simulink model "shortcircuit"  (Simulink 7.6)
settings: Solver=ode45  StartTime=0.0  StopTime=0.2  RelTol=1e-3
libraries: powerlib x10
settings Model: Creator=Martine  LastModifiedBy=ROOTS

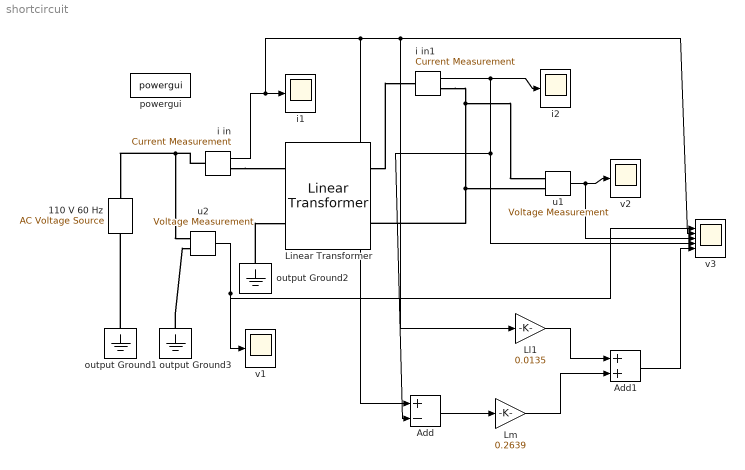
== system shortcircuit ==
  110 V 60 Hz : powerlib/Electrical Sources/AC Voltage Source  Description=source block  DialogController=POWERSYS.PowerSysDialog  SystemSampleTime=-1  Amplitude=155.563  Phase=0  Frequency=60  SampleTime=0  Measurements=None
      settings: AttributesFormatString=\n
  Add : Sum  Inputs=+-
  Add1 : Sum
  Linear Transformer : powerlib/Elements/Linear Transformer  DialogController=POWERSYS.PowerSysDialog  PhysicalDomain=powersysdomain  SubClassName=unknown  LeftPortType=p1  RightPortType=p1  LConnTagsString=a|b  RConnTagsString=A|B  UNITS=SI  NominalPower=[75e3,60]  winding1=[110 6 0.0135]  winding2=[110 5 0.0135]  ThreeWindings=off  winding3=[120 0.00384 0]  RmLm=[99.5 0.2639]  Measurements=None  DataType=on
  Ll1 : Gain  Gain=0.0135
  Lm : Gain  Gain=0.2639
  i in : powerlib/Measurements/Current Measurement  Tag=PoWeRsYsTeMmEaSuReMeNt  DialogController=POWERSYS.PowerSysDialog  SystemSampleTime=-1  PhasorSimulation=off  OutputType=Magnitude  PSBequivalent=0
  i in1 : powerlib/Measurements/Current Measurement  Tag=PoWeRsYsTeMmEaSuReMeNt  DialogController=POWERSYS.PowerSysDialog  SystemSampleTime=-1  PhasorSimulation=off  OutputType=Magnitude  PSBequivalent=0
  i1 : Scope
      settings: DeleteFcn=simscope BlockIsBeingDestroyed  PostSaveFcn=simscope Save  TickLabels=on  TimeRange=0.1  YMin=-10  YMax=10  SaveName=ScopeData3  DataFormat=Array
  i2 : Scope
      settings: DeleteFcn=simscope BlockIsBeingDestroyed  PostSaveFcn=simscope Save  TickLabels=on  TimeRange=0.1  YMin=-12.5  YMax=12.5  SaveName=ScopeData2  DataFormat=Array
  output Ground1 : powerlib/Elements/Ground  DialogController=POWERSYS.PowerSysDialog  PhysicalDomain=powersysdomain  SubClassName=unknown  LeftPortType=p1  RightPortType=p1  LConnTagsString=a
  output Ground2 : powerlib/Elements/Ground  DialogController=POWERSYS.PowerSysDialog  PhysicalDomain=powersysdomain  SubClassName=unknown  LeftPortType=p1  RightPortType=p1  LConnTagsString=a
  output Ground3 : powerlib/Elements/Ground  DialogController=POWERSYS.PowerSysDialog  PhysicalDomain=powersysdomain  SubClassName=unknown  LeftPortType=p1  RightPortType=p1  LConnTagsString=a
  powergui : powerlib/powergui  SystemSampleTime=-1  SimulationMode=Continuous  SampleTime=0  frequency=60  SPID=off  DisableSnubberDevices=off  DisableRonSwitches=off  DisableVfSwitches=off  SwTol=0  Interpol=off  frequencyindice=60  echomessages=off  HookPort=off  DisplayEquations=off  FunctionMessages=off  EnableUseOfTLC=off  x0status=blocks  RestoreLinks=warning  ResistiveCurrentMeasurement=off  Frange=[0:2:500]  Ylog=off  Xlog=on  ShowGrid=off  save=off  variable=ZData  ZoomFFT=on  StartTime=0.0  cycles=1  DisplayStyle=1  fundamental=60  FreqAxis=off  MaxFrequency=1000  frequencyindicesteady=1  RmsSteady=1  display=off  Ts=0  methode=off
  u1 : powerlib/Measurements/Voltage Measurement  Tag=PoWeRsYsTeMmEaSuReMeNt  DialogController=POWERSYS.PowerSysDialog  SystemSampleTime=-1  PhasorSimulation=off  OutputType=Magnitude  PSBequivalent=0
  u2 : powerlib/Measurements/Voltage Measurement  Tag=PoWeRsYsTeMmEaSuReMeNt  DialogController=POWERSYS.PowerSysDialog  SystemSampleTime=-1  PhasorSimulation=off  OutputType=Magnitude  PSBequivalent=0
  v1 : Scope
      settings: DeleteFcn=simscope BlockIsBeingDestroyed  PostSaveFcn=simscope Save  TickLabels=on  TimeRange=0.1  YMin=-200  YMax=200  DataFormat=Array
  v2 : Scope
      settings: DeleteFcn=simscope BlockIsBeingDestroyed  PostSaveFcn=simscope Save  TickLabels=on  TimeRange=0.1  YMin=-200  YMax=200  DataFormat=Array
  v3 : Scope  NumInputPorts=5
      settings: DeleteFcn=simscope BlockIsBeingDestroyed  PostSaveFcn=simscope Save  TickLabels=on  TimeRange=0.2  YMin=-200~-5~-5~-20~-5  YMax=200~5~5~20~5  SaveName=ScopeData4  DataFormat=Array
  wires:
  i in/1 -> i1/1, Add/1, v3/2, Ll1/1
  u1/1 -> v2/1, v3/3
  u2/1 -> v1/1, v3/1
  i in1/1 -> i2/1, v3/4, Add/2
  Add/1 -> Lm/1
  Ll1/1 -> Add1/1
  Lm/1 -> Add1/2
  Add1/1 -> v3/5
  connections:
  i in/LConn1 -- 110 V 60 Hz/RConn1 -- u2/LConn1
  output Ground1/LConn1 -- 110 V 60 Hz/LConn1
  output Ground2/LConn1 -- Linear Transformer/LConn2
  output Ground3/LConn1 -- u2/LConn2
  Linear Transformer/RConn1 -- i in1/LConn1
  i in/RConn1 -- Linear Transformer/LConn1
  i in1/RConn1 -- u1/LConn1 -- Linear Transformer/RConn2 -- u1/LConn2
